simulink model "GRM_Airframe"  (R2018b)
settings: Solver=FixedStepAuto  StartTime=0.0  StopTime=T_sim  FixedStep=0.001  RelTol=1e-3
PreLoadFcn:
  | addpath('init_functions');
  | init_grm;
  | addpath('parameters');
  | para_def_grm;
values from neighbouring files (symbols this model uses):
  act_dmp = 0.6322    [para_def_grm.m]
  act_omega = 59.9250    (= 59.925)    [para_def_grm.m]
  aero = load('aero.mat')    [para_def_grm.m]
  c_be = -6.5e-3    (= -0.0065)    [init_grm.m]
  c_h_geop0 = 0    [init_grm.m]
  c_h_geope = 11e3    (= 11000)    [init_grm.m]
  c_pa0 = 101325    [init_grm.m]
  c_pe = -c_g0/c_be/sgc    (= 5.25587981272)    [init_grm.m]
  c_r0 = 6371000.79    [init_grm.m]
  c_rot = 7.292115e-5    (= 7.292115e-05)    [init_grm.m]
  c_Tmp0 = 288.15    [init_grm.m]
  d_siB_0 = 0    [para_def_grm.m]
  d_siB_max = deg2rad(1200)    [para_def_grm.m]
  d_siB_min = deg2rad(-1200)    [para_def_grm.m]
  dd_siB_max = deg2rad(50000)    [para_def_grm.m]
  dd_siB_min = deg2rad(-50000)    [para_def_grm.m]
  de_JBBB_xx = JBBB_xx_0 - JBBB_xx_e    (= 0)    [para_def_grm.m]
  de_JBBB_yy = JBBB_yy_0 - JBBB_yy_e    (= 0)    [para_def_grm.m]
  de_JBBB_zz = JBBB_zz_0 - JBBB_zz_e    (= 0)    [para_def_grm.m]
  de_mM = m_fuel_lookup(end)    [para_def_grm.m]
  F_prp = [450.52;428.7;423.25;391.61;352.34;304.35;266.17;243.26;216.92 ... (first row only)    [para_def_grm.m]
  flag_I_aero_switch = 1    [init_grm.m]
  flag_I_flat = 1    [init_grm.m]
  flag_I_gravity_switch = 1    [init_grm.m]
  flag_I_rot = 0    [init_grm.m]
  hcr = 1.4    [init_grm.m]
  J0PB_e = TBP*J0PP_e*TBP'    [para_def_grm.m]
  JMMM_0 = TBP*J0PP_0*TBP'    [para_def_grm.m]
  JMMM_e = TBP*J0PP_e*TBP'    [para_def_grm.m]
  lat_0 = 0    [init_grm.m]
  lon_0 = 0    [init_grm.m]
  m0 = mB_0    (= 3.30977)    [para_def_grm.m]
  m_fuel_lookup = [0;0.0573;0.1127;0.1667;0.2186;0.2681;0.3149;0.3588 ... (first row only)    [para_def_grm.m]
  mB_0 = 3.30977    [para_def_grm.m]
  mM_0 = 1.119    [para_def_grm.m]
  mM_e = de_mM    [para_def_grm.m]
  p0PB = [x0PB;y0PB;z0PB]    [para_def_grm.m]
  pBII_0 = TIE_0*pBEE_0    [init_grm.m]
  pMPB = [xMPB;yMPB;zMPB]    [para_def_grm.m]
  pNPB = [0;0;0]    [para_def_grm.m]
  qEG_0 = q12_from_T12(TEG)    [init_grm.m]
  qIB_0 = qumul(qIG_0,qGB_0)    [init_grm.m]
  qIE_0 = q12_from_T12(TIE_0)    [init_grm.m]
  sgc = 287.05287    [init_grm.m]
  siB_0 = 0    [para_def_grm.m]
  siB_max = deg2rad(30)    [para_def_grm.m]
  siB_min = deg2rad(-30)    [para_def_grm.m]
  t_prp1 = [0.04;0.28;0.54;1;1.48;1.99;2.51;3;3.5;3.67;3.82;4]    [para_def_grm.m]
  t_prp2 = t_prp2'    [para_def_grm.m]
  Tr3r4 = [1,1,1,1;1,1,-1,-1;-1,1,1,-1]*0.25    [para_def_grm.m]
  tRRR = 0    [para_def_grm.m]
  unc_act_bl = 0    [para_def_grm.m]
  unc_act_off = 0    [para_def_grm.m]
  unc_act_scale = 1    [para_def_grm.m]
  unc_aero_Cl_scale = 1    [para_def_grm.m]
  unc_aero_Cm_scale = 1    [para_def_grm.m]
  unc_aero_Cn_scale = 1    [para_def_grm.m]
  unc_aero_Cx_scale = 1    [para_def_grm.m]
  unc_aero_Cy_scale = 1    [para_def_grm.m]
  unc_aero_Cz_scale = 1    [para_def_grm.m]
  unc_cg_x = 0    [para_def_grm.m]
  unc_cg_y = 0    [para_def_grm.m]
  unc_cg_z = 0    [para_def_grm.m]
  unc_mB_bl = 0    [para_def_grm.m]
  unc_mB_scale = 1    [para_def_grm.m]
  unc_moi_Jxx = 0    [para_def_grm.m]
  unc_moi_Jyy = 0    [para_def_grm.m]
  unc_moi_Jzz = 0    [para_def_grm.m]
  unc_prp_scale = 1    [para_def_grm.m]
  unc_prp_x = 0    [para_def_grm.m]
  unc_prp_y = 0    [para_def_grm.m]
  unc_prp_z = 0    [para_def_grm.m]
  vBII_0 = vBEE_0 + cross(wIEI_0,pBII_0)    [init_grm.m]
  wBIB_0 = r2_from_r1_trans_q21(wBII_0,qBI_0)    [init_grm.m]
  x0PB = -0.5    [para_def_grm.m]
  xMPB = -0.9    [para_def_grm.m]
  y0PB = 0    [para_def_grm.m]
  yMPB = 0    [para_def_grm.m]
  z0PB = 0    [para_def_grm.m]
  zMPB = 0    [para_def_grm.m]
undefined symbols (not defined in the file or in its folder): c_b_WGS, c_flat, c_grav, c_rsma, d_mB_lookup, t_dmB
libraries: simulink_extras x11, simulink x3
(part 1 of 6)
settings Model: Creator=ga97lot  LastModifiedBy=ga97lot

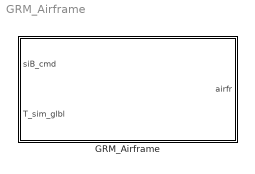
== system GRM_Airframe ==
  GRM_Airframe : Subsystem
      mask Display: image('H:\Sicherung Semesterarbeit\CAD\grm_2.png');

== system GRM_Airframe/GRM_Airframe ==
  siB_cmd : Inport
  T_sim_glbl : Inport  Port=2
  Bus Creator : BusCreator  Inputs=8
  aerodynamics : Subsystem
  environment : Subsystem
  fin_actuators : Subsystem
  forces_moments : Subsystem
  gravity : Subsystem
  input : Subsystem
  motion_kinematics : Subsystem
  propulsion : Subsystem
  rb_eom : Subsystem
  stream_flow : Subsystem
  weight_and_balance : Subsystem
  airfr : Outport
  wires:
  [fin] -> Bus Creator/7
  [motion_kin] -> Bus Creator/6
  [str_flow] -> Bus Creator/5
  [aero] -> Bus Creator/4
  [grav] -> Bus Creator/3
  [prp] -> Bus Creator/8
  [motion_kin] -> rb_eom/1(mot_kin)
  [prp] -> forces_moments/4(prp)
  [motion_kin] -> forces_moments/2(motion_kin)
  Bus Creator/1 -> airfr/1  "airfr_bus"
  [wab] -> Bus Creator/2
  input/1(cmd_bus) -> fin_actuators/1(cmd)
  siB_cmd/1 -> input/1(siB_cmd)
  aerodynamics/1(aero) -> [aero], forces_moments/1(aero)
  forces_moments/1(for_mom_bus) -> rb_eom/2(for_mom)
  stream_flow/1(str_flow) -> [str_flow], aerodynamics/1(str_flow)
  [wab] -> propulsion/2(wab)
  weight_and_balance/1(wab) -> gravity/2(wab), rb_eom/3(wab), [wab]
  T_sim_glbl/1 -> propulsion/1(env_glbl), environment/2(env_glbl), [env_glbl]
  gravity/1(grav) -> forces_moments/3(grav), [grav]
  [env_glbl] -> aerodynamics/4(env_glbl)
  fin_actuators/1(fin) -> aerodynamics/2(fin), [fin]
  [env_glbl] -> weight_and_balance/2(env_glb)
  [wab] -> aerodynamics/3(wab)
  motion_kinematics/1(motion_kin) -> [motion_kin], stream_flow/2(motion_kin)
  propulsion/1(prp) -> [prp], weight_and_balance/1(prp)
  environment/1(env) -> stream_flow/3(env), gravity/1(env)
  rb_eom/1(flight_dyn) -> Bus Creator/1, motion_kinematics/1(flight_dyn), environment/1(flight_dyn), stream_flow/1(flight_dyn)

== system GRM_Airframe/GRM_Airframe/aerodynamics ==
  str_flow : Inport
  fin : Inport  Port=2
  wab : Inport  Port=3
  env_glbl : Inport  Port=4
  Bus Selector : BusSelector  OutputSignals=qdynB,MaB,alB,beB,hBE,wBIB_star
  Bus Selector1 : BusSelector  OutputSignals=afinB
  Bus Selector2 : BusSelector  OutputSignals=pBSB
  aerodynamic_via_lookup : Subsystem
  logic_base_drag : Subsystem
  aero : Outport
  wires:
  logic_base_drag/1(flag_base_drag) -> aerodynamic_via_lookup/9(flag_I_prp)
  env_glbl/1 -> logic_base_drag/1(env_glbl)
  aerodynamic_via_lookup/1(aero_bus) -> aero/1
  Bus Selector/6 -> aerodynamic_via_lookup/7(wBIB_star)  "<wBIB_star>"
  Bus Selector1/1 -> aerodynamic_via_lookup/8(afinB)  "<afinB>"
  Bus Selector/5 -> aerodynamic_via_lookup/6(hBE)  "<hBE>"
  Bus Selector/4 -> aerodynamic_via_lookup/5(beB)  "<beB>"
  Bus Selector/3 -> aerodynamic_via_lookup/4(alB)  "<alB>"
  Bus Selector/2 -> aerodynamic_via_lookup/3(MaB)  "<MaB>"
  Bus Selector/1 -> aerodynamic_via_lookup/2(qdynB)  "<qdynB>"
  Bus Selector2/1 -> aerodynamic_via_lookup/1(pBSB)  "<pBSB>"
  fin/1 -> Bus Selector1/1
  wab/1 -> Bus Selector2/1
  str_flow/1 -> Bus Selector/1

== system GRM_Airframe/GRM_Airframe/environment ==
  flight_dyn : Inport
  env_glbl : Inport  Port=2
  Bus Creator1 : BusCreator  Inputs=2
  Bus Creator2 : BusCreator  Inputs=2
  Bus Selector : BusSelector  OutputSignals=lon,lat,hBE
  Bus Selector1 : BusSelector  OutputSignals=atm_dyn_bus
  Saturation : Saturate  UpperLimit=inf  LowerLimit=eps
      settings: AttributesFormatString=|
      | %<UpperLimit>
      | %<LowerLimit>
  WGS84_Gravitation : Subsystem  mask{flg_omega_enabled=on}
      mask prompts: flg_omega_enabled "Zentripetalbeschleunigung mitberechnen"
      mask help:
      | Dieser Block berechnet die Gravitation für das idealisierte WGS84
      | Ellipsoid. Die Berechnung ist hierbei nach dem Technical Report
      | "Department of Defense World Geodetic System 1984", NIMA TR8350.2,
      | Third Edition, Amendment 1 vom 3 Januar 2000 implementiert.
      | Das Modell ist gültig für alle Höhen über dem WGS84 Referenzellipsoid, und
      | ist somit der reinen Taylorexpansion des Somigliana Modells überlegen
      | (siehe Kapitel 4.3 des WGS84 reports).
      |
      | ---------------------------------------------------------------------------
      | Longitude [rad]: Nach WGS84 definierte Geodätische Länge.  (lambda)
      | Lattitude [rad]: Nach WGS84 definierte Geodätische Breite. (phi)
      | Height [m]: Höhe über dem WGS84 Referenzellipsoid.
      mask init:
      | [ c_rsma, c_b_WGS, c_grav, c_rot] = init_WGS84_Gravitationsmodell();
  atmosphere_static_ISO_2533 : Subsystem
  convert_to_local_frame : Subsystem
  env : Outport
  wires:
  Bus Selector1/1 -> Bus Creator1/2  "<atm_dyn_bus>"
  env_glbl/1 -> atmosphere_static_ISO_2533/2(env_glbl), Bus Selector1/1
  atmosphere_static_ISO_2533/1(atm_stat) -> Bus Creator1/1  "atm_stat_bus"
  Saturation/1 -> WGS84_Gravitation/3(h)
  Bus Creator1/1 -> Bus Creator2/2  "atm_bus"
  Bus Selector/2 -> WGS84_Gravitation/2(lat)  "<lat>"
  Bus Creator2/1 -> env/1  "env_bus"
  Bus Selector/3 -> Saturation/1, atmosphere_static_ISO_2533/1(hBE)  "<hBE>"
  Bus Selector/1 -> WGS84_Gravitation/1(lon)  "<lon>"
  WGS84_Gravitation/1(gE) -> convert_to_local_frame/1(gE)
  flight_dyn/1 -> Bus Selector/1
  convert_to_local_frame/1(gBG) -> Bus Creator2/1

== system GRM_Airframe/GRM_Airframe/fin_actuators ==
  cmd : Inport
  Bus Creator3 : BusCreator  Inputs=7
  Bus Selector : BusSelector  OutputSignals=siB_cmd
  Constant7 : Constant  Value=tRRR
  Demux : Demux
  Rudder : Subsystem  mask{siB_max=siB_max, siB_min=siB_min, d_siB_max=d_siB_max, d_siB_min=d_siB_min, dd_siB_max=dd_siB_max, dd_siB_min=dd_siB_min, omega=act_omega, dmp=act_dmp, unc_bl=unc_act_bl, unc_scale=unc_act_scale, unc_off=unc_act_off, siB_0=siB_0, d_siB_0=d_siB_0}
      mask prompts: siB_max "Obere Limitierung des Ruderstellwinkels in [rad]"; siB_min "Untere Limitierung des Ruderstellwinkels in [rad]"; d_siB_max "Obere Limitierung der Ruderstellwinkelgeschwindigkeit in [rad/s]"; d_siB_min "Untere Limitierung der Ruderstellwinkelgeschwindigkeit in [rad/s]"; dd_siB_max "Obere Limitierung der Ruderstellwinkelbeschleunigung in [rad/s^2]"; dd_siB_min "Untere Limitierung der Ruderstellwinkelbeschleunigung in [rad/s^2]"; omega "Eckfrequenz in [Hz]"; dmp "Dämpfung in [kg/s]"; unc_bl "Rückschlag des Aktuators (Backlash) in [rad]"; unc_scale "Skalenfehler in [-]"; unc_off "Versatz (Offset) in [rad]"; siB_0 "Startwert Ruderwinkel in [rad]"; d_siB_0 "Startwert Ruderwinkelgeschwindigkeiten in [rad/s]"
      mask DialogControl ParameterGroupVar Prompt: Limitierungen
      mask DialogControl Container3 Prompt: Dynamik
      mask DialogControl Container4 Prompt: Aktuatorfehler
      mask DialogControl Container5 Prompt: Startwerte
  Rudder1 : Subsystem  mask{siB_max=siB_max, siB_min=siB_min, d_siB_max=d_siB_max, d_siB_min=d_siB_min, dd_siB_max=dd_siB_max, dd_siB_min=dd_siB_min, omega=act_omega, dmp=act_dmp, unc_bl=unc_act_bl, unc_scale=unc_act_scale, unc_off=unc_act_off, siB_0=siB_0, d_siB_0=d_siB_0}
      mask prompts: siB_max "Obere Limitierung des Ruderstellwinkels in [rad]"; siB_min "Untere Limitierung des Ruderstellwinkels in [rad]"; d_siB_max "Obere Limitierung der Ruderstellwinkelgeschwindigkeit in [rad/s]"; d_siB_min "Untere Limitierung der Ruderstellwinkelgeschwindigkeit in [rad/s]"; dd_siB_max "Obere Limitierung der Ruderstellwinkelbeschleunigung in [rad/s^2]"; dd_siB_min "Untere Limitierung der Ruderstellwinkelbeschleunigung in [rad/s^2]"; omega "Eckfrequenz in [Hz]"; dmp "Dämpfung in [kg/s]"; unc_bl "Rückschlag des Aktuators (Backlash) in [rad]"; unc_scale "Skalenfehler in [-]"; unc_off "Versatz (Offset) in [rad]"; siB_0 "Startwert Ruderwinkel in [rad]"; d_siB_0 "Startwert Ruderwinkelgeschwindigkeiten in [rad/s]"
      mask DialogControl ParameterGroupVar Prompt: Limitierungen
      mask DialogControl Container3 Prompt: Dynamik
      mask DialogControl Container4 Prompt: Aktuatorfehler
      mask DialogControl Container5 Prompt: Startwerte
  Rudder2 : Subsystem  mask{siB_max=siB_max, siB_min=siB_min, d_siB_max=d_siB_max, d_siB_min=d_siB_min, dd_siB_max=dd_siB_max, dd_siB_min=dd_siB_min, omega=act_omega, dmp=act_dmp, unc_bl=unc_act_bl, unc_scale=unc_act_scale, unc_off=unc_act_off, siB_0=siB_0, d_siB_0=d_siB_0}
      mask prompts: siB_max "Obere Limitierung des Ruderstellwinkels in [rad]"; siB_min "Untere Limitierung des Ruderstellwinkels in [rad]"; d_siB_max "Obere Limitierung der Ruderstellwinkelgeschwindigkeit in [rad/s]"; d_siB_min "Untere Limitierung der Ruderstellwinkelgeschwindigkeit in [rad/s]"; dd_siB_max "Obere Limitierung der Ruderstellwinkelbeschleunigung in [rad/s^2]"; dd_siB_min "Untere Limitierung der Ruderstellwinkelbeschleunigung in [rad/s^2]"; omega "Eckfrequenz in [Hz]"; dmp "Dämpfung in [kg/s]"; unc_bl "Rückschlag des Aktuators (Backlash) in [rad]"; unc_scale "Skalenfehler in [-]"; unc_off "Versatz (Offset) in [rad]"; siB_0 "Startwert Ruderwinkel in [rad]"; d_siB_0 "Startwert Ruderwinkelgeschwindigkeiten in [rad/s]"
      mask DialogControl ParameterGroupVar Prompt: Limitierungen
      mask DialogControl Container3 Prompt: Dynamik
      mask DialogControl Container4 Prompt: Aktuatorfehler
      mask DialogControl Container5 Prompt: Startwerte
  Rudder3 : Subsystem  mask{siB_max=siB_max, siB_min=siB_min, d_siB_max=d_siB_max, d_siB_min=d_siB_min, dd_siB_max=dd_siB_max, dd_siB_min=dd_siB_min, omega=act_omega, dmp=act_dmp, unc_bl=unc_act_bl, unc_scale=unc_act_scale, unc_off=unc_act_off, siB_0=siB_0, d_siB_0=d_siB_0}
      mask prompts: siB_max "Obere Limitierung des Ruderstellwinkels in [rad]"; siB_min "Untere Limitierung des Ruderstellwinkels in [rad]"; d_siB_max "Obere Limitierung der Ruderstellwinkelgeschwindigkeit in [rad/s]"; d_siB_min "Untere Limitierung der Ruderstellwinkelgeschwindigkeit in [rad/s]"; dd_siB_max "Obere Limitierung der Ruderstellwinkelbeschleunigung in [rad/s^2]"; dd_siB_min "Untere Limitierung der Ruderstellwinkelbeschleunigung in [rad/s^2]"; omega "Eckfrequenz in [Hz]"; dmp "Dämpfung in [kg/s]"; unc_bl "Rückschlag des Aktuators (Backlash) in [rad]"; unc_scale "Skalenfehler in [-]"; unc_off "Versatz (Offset) in [rad]"; siB_0 "Startwert Ruderwinkel in [rad]"; d_siB_0 "Startwert Ruderwinkelgeschwindigkeiten in [rad/s]"
      mask DialogControl ParameterGroupVar Prompt: Limitierungen
      mask DialogControl Container3 Prompt: Dynamik
      mask DialogControl Container4 Prompt: Aktuatorfehler
      mask DialogControl Container5 Prompt: Startwerte
  Vector Concatenate1 : Concatenate  NumInputs=4
  Vector Concatenate2 : Concatenate  NumInputs=4
  Vector Concatenate3 : Concatenate  NumInputs=4
  control_allocation : Subsystem
  fin : Outport
  wires:
  control_allocation/4(dd_finB) -> Bus Creator3/5
  control_allocation/3(d_finB) -> Bus Creator3/4
  control_allocation/2(finB) -> Bus Creator3/3
  control_allocation/1(Tr3r4) -> Bus Creator3/2
  Vector Concatenate3/1 -> control_allocation/3(dd_siB), Bus Creator3/6  "dd_siB"
  Vector Concatenate2/1 -> control_allocation/2(d_siB), Bus Creator3/7  "d_siB"
  Vector Concatenate1/1 -> control_allocation/1(siB), Bus Creator3/1  "siB"
  Bus Creator3/1 -> fin/1  "fin_bus"
  Rudder/1(siB) -> Vector Concatenate1/1
  Rudder/3(dd_siB) -> [dd_siB1]
  Demux/2 -> Rudder1/1(siB_c)
  Rudder2/3(dd_siB) -> [dd_siB3]
  Rudder/2(d_siB) -> [d_siB1]
  Rudder3/3(dd_siB) -> [dd_siB4]
  Rudder1/3(dd_siB) -> [dd_siB2]
  Rudder1/1(siB) -> Vector Concatenate1/2
  [dd_siB1] -> Vector Concatenate3/1
  cmd/1 -> Bus Selector/1
  [dd_siB3] -> Vector Concatenate3/3
  [dd_siB4] -> Vector Concatenate3/4
  Demux/1 -> Rudder/1(siB_c)
  Rudder3/2(d_siB) -> [d_siB4]
  Demux/3 -> Rudder2/1(siB_c)
  [dd_siB2] -> Vector Concatenate3/2
  Constant7/1 -> Rudder/2(tRRR), Rudder2/2(tRRR), Rudder3/2(tRRR), Rudder1/2(tRRR)
  [d_siB2] -> Vector Concatenate2/2
  Bus Selector/1 -> Demux/1  "<siB_cmd>"
  [d_siB1] -> Vector Concatenate2/1
  [d_siB4] -> Vector Concatenate2/4
  Rudder2/1(siB) -> Vector Concatenate1/3
  Rudder1/2(d_siB) -> [d_siB2]
  Rudder3/1(siB) -> Vector Concatenate1/4
  Rudder2/2(d_siB) -> [d_siB3]
  Demux/4 -> Rudder3/1(siB_c)
  [d_siB3] -> Vector Concatenate2/3

== system GRM_Airframe/GRM_Airframe/forces_moments ==
  aero : Inport
  motion_kin : Inport  Port=2
  grav : Inport  Port=3
  prp : Inport  Port=4
  Add : Sum  Inputs=+++
  Add1 : Sum
  Bus Creator : BusCreator  Inputs=2
  Bus Selector : BusSelector  OutputSignals=FBAB,MBAB
  Bus Selector1 : BusSelector  OutputSignals=TGB
  Bus Selector2 : BusSelector  OutputSignals=FBGG
  Bus Selector3 : BusSelector  OutputSignals=FBPB,MBPB
  Math Function : Math  Operator=transpose  SaturateOnIntegerOverflow=on
  Product : Product  Multiplication=Matrix(*)
  for_mom_bus : Outport
  wires:
  Bus Selector3/2 -> Add1/2  "<MBPB>"
  Bus Creator/1 -> for_mom_bus/1  "for_mom_bus"
  Bus Selector3/1 -> Add/3  "<FBPB>"
  Bus Selector/2 -> Add1/1  "<MBAB>"
  Add1/1 -> Bus Creator/2  "MBTB"
  grav/1 -> Bus Selector2/1
  Add/1 -> Bus Creator/1  "FBTB"
  motion_kin/1 -> Bus Selector1/1
  prp/1 -> Bus Selector3/1
  Product/1 -> Add/2  "FBGB"
  aero/1 -> Bus Selector/1
  Math Function/1 -> Product/1  "TBG"
  Bus Selector1/1 -> Math Function/1  "<TGB>"
  Bus Selector2/1 -> Product/2  "<FBGG>"
  Bus Selector/1 -> Add/1  "<FBAB>"

== system GRM_Airframe/GRM_Airframe/gravity ==
  env : Inport
  wab : Inport  Port=2
  Bus Creator3 : BusCreator  Inputs=1
  Bus Selector : BusSelector  OutputSignals=gBG,atm_bus.atm_stat_bus.hBE
  Bus Selector1 : BusSelector  OutputSignals=mB
  Product : Product
  launch_rail : Subsystem
  grav : Outport
  wires:
  env/1 -> Bus Selector/1
  Bus Selector1/1 -> Product/2  "<mB>"
  wab/1 -> Bus Selector1/1
  Bus Creator3/1 -> grav/1  "grav_bus"
  Product/1 -> Bus Creator3/1  "FBGG"
  Bus Selector/1 -> launch_rail/1(gBG_c)  "<gBG>"
  Bus Selector/2 -> launch_rail/2(hBE)  "<hBE>"
  launch_rail/1(gBG) -> Product/1

== system GRM_Airframe/GRM_Airframe/input ==
  siB_cmd : Inport
  Bus Creator2 : BusCreator  Inputs=1
  cmd_bus : Outport
  wires:
  Bus Creator2/1 -> cmd_bus/1  "cmd_bus"
  siB_cmd/1 -> Bus Creator2/1

== system GRM_Airframe/GRM_Airframe/motion_kinematics ==
  flight_dyn : Inport
  Bus Creator : BusCreator  Inputs=7
  Bus Selector : BusSelector  OutputSignals=lat,lon,qIB
  calc_motion_kinematics : Subsystem
  motion_kin : Outport
  wires:
  calc_motion_kinematics/7(TIB) -> Bus Creator/7
  calc_motion_kinematics/6(wEGG) -> Bus Creator/6
  calc_motion_kinematics/5(TEG) -> Bus Creator/5
  calc_motion_kinematics/4(TGB) -> Bus Creator/4
  calc_motion_kinematics/3(TEB) -> Bus Creator/3
  calc_motion_kinematics/2(TIE) -> Bus Creator/2
  calc_motion_kinematics/1(wIEE) -> Bus Creator/1
  Bus Selector/3 -> calc_motion_kinematics/3(qIB)  "<qIB>"
  Bus Selector/2 -> calc_motion_kinematics/2(lon)  "<lon>"
  Bus Selector/1 -> calc_motion_kinematics/1(lat)  "<lat>"
  Bus Creator/1 -> motion_kin/1  "motion_kin_bus"
  flight_dyn/1 -> Bus Selector/1

== system GRM_Airframe/GRM_Airframe/propulsion ==
  env_glbl : Inport
  wab : Inport  Port=2
  Bus Creator1 : BusCreator  Inputs=3
  prp_look_up : Subsystem
  prp_uncertainty : Subsystem
  prp : Outport
  wires:
  prp_look_up/1(dmB) -> Bus Creator1/1
  wab/1 -> prp_uncertainty/2(wab)
  prp_uncertainty/1(FBPB) -> Bus Creator1/2
  prp_uncertainty/2(MBPB) -> Bus Creator1/3
  env_glbl/1 -> prp_look_up/1(env_glbl_bus)
  prp_look_up/2(FBPM) -> prp_uncertainty/1(FBPM)
  Bus Creator1/1 -> prp/1  "prp_bus"

== system GRM_Airframe/GRM_Airframe/rb_eom ==
  mot_kin : Inport
  for_mom : Inport  Port=2
  wab : Inport  Port=3
  Bus Creator : BusCreator  Inputs=12
  calc_bus_flight_dyn_bus_entries : Subsystem
  eom_6dof : Subsystem
  flight_dyn : Outport
  wires:
  calc_bus_flight_dyn_bus_entries/12(vBIB) -> Bus Creator/12
  calc_bus_flight_dyn_bus_entries/11(euIB) -> Bus Creator/11
  calc_bus_flight_dyn_bus_entries/10(pBII) -> Bus Creator/10
  eom_6dof/1(eom) -> calc_bus_flight_dyn_bus_entries/2(eom)
  wab/1 -> eom_6dof/2(wab)
  for_mom/1 -> eom_6dof/1(for_mom)
  Bus Creator/1 -> flight_dyn/1  "flight_dyn_bus"
  calc_bus_flight_dyn_bus_entries/9(d_vBII) -> Bus Creator/9
  calc_bus_flight_dyn_bus_entries/8(d_wBIB) -> Bus Creator/8
  calc_bus_flight_dyn_bus_entries/7(wBIB) -> Bus Creator/7
  calc_bus_flight_dyn_bus_entries/6(qIB) -> Bus Creator/6
  calc_bus_flight_dyn_bus_entries/5(vBII) -> Bus Creator/5
  calc_bus_flight_dyn_bus_entries/4(hBE) -> Bus Creator/4
  calc_bus_flight_dyn_bus_entries/3(lat) -> Bus Creator/3
  calc_bus_flight_dyn_bus_entries/2(lon) -> Bus Creator/2
  calc_bus_flight_dyn_bus_entries/1(aBIB) -> Bus Creator/1
  mot_kin/1 -> calc_bus_flight_dyn_bus_entries/1(mot_kin)

== system GRM_Airframe/GRM_Airframe/stream_flow ==
  flight_dyn : Inport
  motion_kin : Inport  Port=2
  env : Inport  Port=3
  Bus Selector1 : BusSelector  OutputSignals=atm_bus.atm_stat_bus.rho,atm_bus.atm_stat_bus.sos,atm_bus.atm_stat_bus.hBE,atm_bus.atm_dyn_bus.vWEG
  Bus Selector2 : BusSelector  OutputSignals=vBII,pBII,wBIB
  Bus Selector3 : BusSelector  OutputSignals=TIB,wIEE,TIE,TGB
  calc_stream_flow : Subsystem
  str_flow : Outport
  wires:
  Bus Selector3/4 -> calc_stream_flow/4(TGB)  "<TGB>"
  Bus Selector1/4 -> calc_stream_flow/11(vWEG)  "<vWEG>"
  Bus Selector2/2 -> calc_stream_flow/6(pBII)  "<pBII>"
  calc_stream_flow/1(str_flow) -> str_flow/1
  Bus Selector1/3 -> calc_stream_flow/10(hBE)  "<hBE>"
  Bus Selector1/2 -> calc_stream_flow/9(sos)  "<sos>"
  Bus Selector1/1 -> calc_stream_flow/8(rho)  "<rho>"
  Bus Selector2/3 -> calc_stream_flow/7(wBIB)  "<wBIB>"
  Bus Selector2/1 -> calc_stream_flow/5(vBII)  "<vBII>"
  Bus Selector3/3 -> calc_stream_flow/3(TIE)  "<TIE>"
  Bus Selector3/2 -> calc_stream_flow/2(wIEE)  "<wIEE>"
  Bus Selector3/1 -> calc_stream_flow/1(TIB)  "<TIB>"
  env/1 -> Bus Selector1/1
  flight_dyn/1 -> Bus Selector2/1
  motion_kin/1 -> Bus Selector3/1

== system GRM_Airframe/GRM_Airframe/weight_and_balance ==
  prp : Inport
  env_glb : Inport  Port=2
  Bus Creator1 : BusCreator  Inputs=4
  Bus Selector2 : BusSelector  OutputSignals=T_sim_glbl,T_sim_lnch
  Subtract : Sum  Inputs=+-
  center_of_gravity : Subsystem
  d_moi : Subsystem
  mass : Subsystem
  mass_uncertainty : Subsystem
  moi : Subsystem
  wab : Outport
  wires:
  d_moi/1(d_JBBB) -> Bus Creator1/4
  prp/1 -> d_moi/1(prp)
  Subtract/1 -> mass/1(sim_time_launch)
  mass/1(mB_c) -> mass_uncertainty/1(mB_c)
  mass_uncertainty/1(mB) -> Bus Creator1/1, center_of_gravity/1(mB)
  mass/2(mM) -> center_of_gravity/2(mM), moi/2(mM)
  moi/1(JBBB) -> Bus Creator1/3
  center_of_gravity/1(pBSB) -> Bus Creator1/2, moi/1(pBPB)
  Bus Creator1/1 -> wab/1  "wab_bus"
  env_glb/1 -> Bus Selector2/1
  Bus Selector2/1 -> Subtract/1  "<T_sim_glbl>"
  Bus Selector2/2 -> Subtract/2  "<T_sim_lnch>"

== system GRM_Airframe/GRM_Airframe/aerodynamics/aerodynamic_via_lookup ==
  pBSB : Inport
  qdynB : Inport  Port=2
  MaB : Inport  Port=3
  alB : Inport  Port=4
  beB : Inport  Port=5
  hBE : Inport  Port=6
  wBIB_star : Inport  Port=7
  afinB : Inport  Port=8
  flag_I_prp : Inport  Port=9
  Bus Creator : BusCreator  Inputs=2
  calc_aero_coefficients : Subsystem
  calc_aero_for_mom : Subsystem
  calc_derivatives : Subsystem
  transform_rad2deg_al_be : Subsystem
  transform_rad2deg_fin : Subsystem
  transform_rad2deg_rates : Subsystem
  aero_bus : Outport
  wires:
  transform_rad2deg_al_be/2(beB_deg) -> calc_derivatives/4(beB)
  transform_rad2deg_al_be/1(alB_deg) -> calc_derivatives/3(alB)
  beB/1 -> transform_rad2deg_al_be/2(beB)
  afinB/1 -> transform_rad2deg_fin/1(afinB)
  qdynB/1 -> calc_aero_for_mom/3(qdynB)
  calc_aero_for_mom/2(MBAB) -> Bus Creator/2
  calc_aero_coefficients/6(Cn) -> calc_aero_for_mom/9(Cn)
  calc_aero_coefficients/1(Cx) -> calc_aero_for_mom/4(Cx)
  calc_aero_coefficients/5(Cm) -> calc_aero_for_mom/8(Cm)
  calc_derivatives/4(Cl_deriv) -> calc_aero_coefficients/4(Cl_deriv)
  calc_aero_coefficients/3(Cz) -> calc_aero_for_mom/6(Cz)
  hBE/1 -> calc_aero_for_mom/1(hBE), calc_derivatives/1(hBE)
  flag_I_prp/1 -> calc_aero_coefficients/13(flag_base_drag)
  calc_derivatives/6(Cn_deriv) -> calc_aero_coefficients/6(Cn_deriv)
  wBIB_star/1 -> transform_rad2deg_rates/1(wBIB_star)
  calc_derivatives/3(Cz_deriv) -> calc_aero_coefficients/3(Cz_deriv)
  pBSB/1 -> calc_aero_for_mom/2(pBSB)
  transform_rad2deg_rates/2(qBIB_star_deg) -> calc_aero_coefficients/11(qBIB_star)
  transform_rad2deg_rates/3(rBIB_star_deg) -> calc_aero_coefficients/12(rBIB_star)
  Bus Creator/1 -> aero_bus/1  "aero_bus"
  calc_aero_coefficients/2(Cy) -> calc_aero_for_mom/5(Cy)
  calc_derivatives/5(Cm_deriv) -> calc_aero_coefficients/5(Cm_deriv)
  calc_derivatives/2(Cy_deriv) -> calc_aero_coefficients/2(Cy_deriv)
  transform_rad2deg_rates/1(pBIB_star_deg) -> calc_aero_coefficients/10(pBIB_star)
  transform_rad2deg_fin/3(xiB_deg) -> calc_aero_coefficients/9(xiB_deg)
  transform_rad2deg_fin/2(zeB_deg) -> calc_aero_coefficients/8(zeB_deg), calc_derivatives/6(zeB_deg)
  alB/1 -> transform_rad2deg_al_be/1(alB)
  transform_rad2deg_fin/1(etB_deg) -> calc_derivatives/5(etB_deg), calc_aero_coefficients/7(etB_deg)
  calc_derivatives/1(Cx_deriv) -> calc_aero_coefficients/1(Cx_deriv)
  calc_aero_for_mom/1(FBAB) -> Bus Creator/1
  MaB/1 -> calc_derivatives/2(MaB)
  calc_aero_coefficients/4(Cl) -> calc_aero_for_mom/7(Cl)

== system GRM_Airframe/GRM_Airframe/aerodynamics/logic_base_drag ==
  env_glbl : Inport
  Bus Selector1 : BusSelector  OutputSignals=T_sim_glbl,T_sim_lnch
  Constant : Constant  Value=t_prp2(end)
  MATLAB Function : MATLAB Function  TreatAsAtomicUnit=on
  Subtract : Sum  Inputs=+-
  flag_base_drag : Outport
  wires:
  env_glbl/1 -> Bus Selector1/1
  Bus Selector1/2 -> Subtract/2  "<T_sim_lnch>"
  Bus Selector1/1 -> Subtract/1  "<T_sim_glbl>"
  MATLAB Function/1(flag_base_drag) -> flag_base_drag/1  "flag_base_drag"
  Constant/1 -> MATLAB Function/2(t_prp2)
  Subtract/1 -> MATLAB Function/1(u)

== system GRM_Airframe/GRM_Airframe/environment/WGS84_Gravitation ==
  lon : Inport  PortDimensions=1
  lat : Inport  Port=2  PortDimensions=1
  h : Inport  Port=3  PortDimensions=1
  Assertion : Assertion  AssertionFailFcn="error('WGS84 Gravitationsmodell: Die Werte des Eingangs \"h\" muessen groesser als 0 sein')"
  Assertion1 : Assertion  AssertionFailFcn="error('WGS84 Gravitationsmodell: Die Werte des Eingangs \"Long\" muessen zwischen -180 und +180 liegen')"
  Assertion2 : Assertion  AssertionFailFcn="error('WGS84 Gravitationsmodell: Die Werte des Eingangs \"Lat\" muessen zwischen -90 und +90 liegen')"
  Compare To Constant : simulink/Logic and Bit Operations/Compare To Constant  relop=>=  const=0  OutDataTypeStr=boolean
      settings: SourceProductName=ISim Simulink Block Set
  Interval Test : simulink/Logic and Bit Operations/Interval Test  IntervalClosedRight=on  uplimit=pi  IntervalClosedLeft=on  lowlimit=-pi  OutDataTypeStr=boolean
      settings: SourceProductName=ISim Simulink Block Set
  Interval Test1 : simulink/Logic and Bit Operations/Interval Test  IntervalClosedRight=on  uplimit=pi/2  IntervalClosedLeft=on  lowlimit=-pi/2  OutDataTypeStr=boolean
      settings: SourceProductName=ISim Simulink Block Set
  WGS84_2_ECEF : Subsystem
  WGS84_Gravity_Implementation : MATLAB Function  TreatAsAtomicUnit=on
  gE : Outport  PortDimensions=3
  wires:
  WGS84_Gravity_Implementation/1(gamma_R) -> gE/1  "gE"
  h/1 -> Compare To Constant/1, WGS84_2_ECEF/1(h)  "h"
  lon/1 -> WGS84_2_ECEF/2(lon), Interval Test/1, WGS84_Gravity_Implementation/3(long_rad)  "lon"
  lat/1 -> WGS84_2_ECEF/3(lat), Interval Test1/1, WGS84_Gravity_Implementation/2(lat_rad)  "lat"
  WGS84_2_ECEF/1(pE) -> WGS84_Gravity_Implementation/1(pE)  "pE"
  Compare To Constant/1 -> Assertion/1
  Interval Test/1 -> Assertion1/1
  Interval Test1/1 -> Assertion2/1

== system GRM_Airframe/GRM_Airframe/environment/atmosphere_static_ISO_2533 ==
  hBE : Inport
  env_glbl : Inport  Port=2
  Bus Creator1 : BusCreator  Inputs=6
  Bus Selector1 : BusSelector  OutputSignals=e_Tmp,e_pa
  Saturation : Saturate  UpperLimit=c_h_geope  LowerLimit=c_h_geop0
      settings: AttributesFormatString=|
      | %<UpperLimit>
      | %<LowerLimit>
  density : Subsystem
  geopot_height : Subsystem  mask{mean_earth_radius=c_r0}
      mask prompts: mean_earth_radius "Mean Earth Radius WGS 84 [m]"
      mask TypeOptions mean_earth_radius: mean_earth_radius/Value
  speed_of_sound : Subsystem
  tmp_and_pressure_ISO_2533 : Subsystem
  atm_stat : Outport
  wires:
  Saturation/1 -> tmp_and_pressure_ISO_2533/1(h_geop), Bus Creator1/2  "h_geop"
  hBE/1 -> geopot_height/1(hBE), Bus Creator1/1
  density/1(rho) -> Bus Creator1/5
  tmp_and_pressure_ISO_2533/2(pa) -> density/2(pa), Bus Creator1/6
  tmp_and_pressure_ISO_2533/1(Tmp) -> density/1(Tmp), Bus Creator1/4, speed_of_sound/1(Tmp)
  Bus Creator1/1 -> atm_stat/1  "atm_stat_bus"
  Bus Selector1/1 -> tmp_and_pressure_ISO_2533/2(e_Tmp)  "<e_Tmp>"
  geopot_height/1(h_geop) -> Saturation/1
  Bus Selector1/2 -> tmp_and_pressure_ISO_2533/3(e_pa)  "<e_pa>"
  env_glbl/1 -> Bus Selector1/1
  speed_of_sound/1(sos) -> Bus Creator1/3

== system GRM_Airframe/GRM_Airframe/environment/convert_to_local_frame ==
  gE : Inport
  Constant1 : Constant  Value=0
  Dot Product : DotProduct  InputSameDT=on  OutDataTypeStr=Inherit: Inherit via internal rule
  Sqrt : Sqrt  SaturateOnIntegerOverflow=on
  Vector Concatenate : Concatenate  NumInputs=3  Mode=Multidimensional array
  gBG : Outport
  wires:
  Dot Product/1 -> Sqrt/1
  Vector Concatenate/1 -> gBG/1  "gBG"
  Sqrt/1 -> Vector Concatenate/3
  Constant1/1 -> Vector Concatenate/1, Vector Concatenate/2
  gE/1 -> Dot Product/2, Dot Product/1

== system GRM_Airframe/GRM_Airframe/fin_actuators/Rudder ==
  siB_c : Inport
  tRRR : Inport  Port=2
  Add : Sum  Inputs=+-
  Add1 : Sum  Inputs=+-
  Add2 : Sum  Inputs=+++
  Constant : Constant  Value=unc_off
  Gain : Gain  Gain=omega^2
  Gain1 : Gain  Gain=unc_scale
  Gain2 : Gain  Gain=2*dmp*omega  Multiplication=Matrix(K*u)
  Gain3 : Gain  Gain=unc_bl
  Integrator : Integrator  ExternalReset=either  InitialCondition=d_siB_0
  Integrator1 : Integrator  InitialCondition=siB_0  LimitOutput=on  UpperSaturationLimit=siB_max  LowerSaturationLimit=siB_min  ShowSaturationPort=on
  Limiting_Acceleration : MATLAB Function  TreatAsAtomicUnit=on
  Limiting_Rate : MATLAB Function  TreatAsAtomicUnit=on
  Saturation : Saturate  UpperLimit=siB_max  LowerLimit=siB_min
  Saturation1 : Saturate  UpperLimit=siB_max  LowerLimit=siB_min
  Sign : Signum
  siB : Outport
  d_siB : Outport  Port=2
  dd_siB : Outport  Port=3
  wires:
  [siB] -> Limiting_Rate/1(siB)
  [siB] -> Limiting_Acceleration/1(siB)
  [d_siB] -> Limiting_Acceleration/2(d_siB)
  siB_c/1 -> Saturation/1  "siB_c"
  Constant/1 -> Add2/1
  Add2/1 -> Saturation1/1
  Saturation/1 -> Add/1
  Integrator/1 -> Gain2/1, Limiting_Rate/2(d_siB)  "d_siB"
  Limiting_Rate/1(d_siB_l) -> Integrator1/1, [d_siB], d_siB/1  "d_siB_l"
  Limiting_Acceleration/1(dd_siB_l) -> dd_siB/1, Integrator/1  "dd_siB_l"
  Add/1 -> Gain/1
  Gain/1 -> Add1/1
  Gain2/1 -> Add1/2
  Add1/1 -> Limiting_Acceleration/3(dd_siB)  "dd_siB"
  Integrator1/1 -> Add/2, Gain1/1  "siB"
  tRRR/1 -> Sign/1  "tRRR"
  Sign/1 -> Gain3/1
  Gain3/1 -> Add2/3
  Gain1/1 -> Add2/2
  Integrator1/2 -> Integrator/2  "sat"
  Saturation1/1 -> [siB], siB/1  "siB"

== system GRM_Airframe/GRM_Airframe/fin_actuators/Rudder1 ==
  siB_c : Inport
  tRRR : Inport  Port=2
  Add : Sum  Inputs=+-
  Add1 : Sum  Inputs=+-
  Add2 : Sum  Inputs=+++
  Constant : Constant  Value=unc_off
  Gain : Gain  Gain=omega^2
  Gain1 : Gain  Gain=unc_scale
  Gain2 : Gain  Gain=2*dmp*omega  Multiplication=Matrix(K*u)
  Gain3 : Gain  Gain=unc_bl
  Integrator : Integrator  ExternalReset=either  InitialCondition=d_siB_0
  Integrator1 : Integrator  InitialCondition=siB_0  LimitOutput=on  UpperSaturationLimit=siB_max  LowerSaturationLimit=siB_min  ShowSaturationPort=on
  Limiting_Acceleration : MATLAB Function  TreatAsAtomicUnit=on
  Limiting_Rate : MATLAB Function  TreatAsAtomicUnit=on
  Saturation : Saturate  UpperLimit=siB_max  LowerLimit=siB_min
  Saturation1 : Saturate  UpperLimit=siB_max  LowerLimit=siB_min
  Sign : Signum
  siB : Outport
  d_siB : Outport  Port=2
  dd_siB : Outport  Port=3
  wires:
  [siB] -> Limiting_Rate/1(siB)
  [siB] -> Limiting_Acceleration/1(siB)
  [d_siB] -> Limiting_Acceleration/2(d_siB)
  siB_c/1 -> Saturation/1  "siB_c"
  Constant/1 -> Add2/1
  Add2/1 -> Saturation1/1
  Saturation/1 -> Add/1
  Integrator/1 -> Gain2/1, Limiting_Rate/2(d_siB)  "d_siB"
  Limiting_Rate/1(d_siB_l) -> Integrator1/1, [d_siB], d_siB/1  "d_siB_l"
  Limiting_Acceleration/1(dd_siB_l) -> dd_siB/1, Integrator/1  "dd_siB_l"
  Add/1 -> Gain/1
  Gain/1 -> Add1/1
  Gain2/1 -> Add1/2
  Add1/1 -> Limiting_Acceleration/3(dd_siB)  "dd_siB"
  Integrator1/1 -> Add/2, Gain1/1  "siB"
  tRRR/1 -> Sign/1  "tRRR"
  Sign/1 -> Gain3/1
  Gain3/1 -> Add2/3
  Gain1/1 -> Add2/2
  Integrator1/2 -> Integrator/2  "sat"
  Saturation1/1 -> [siB], siB/1  "siB"

== system GRM_Airframe/GRM_Airframe/fin_actuators/Rudder2 ==
  siB_c : Inport
  tRRR : Inport  Port=2
  Add : Sum  Inputs=+-
  Add1 : Sum  Inputs=+-
  Add2 : Sum  Inputs=+++
  Constant : Constant  Value=unc_off
  Gain : Gain  Gain=omega^2
  Gain1 : Gain  Gain=unc_scale
  Gain2 : Gain  Gain=2*dmp*omega  Multiplication=Matrix(K*u)
  Gain3 : Gain  Gain=unc_bl
  Integrator : Integrator  ExternalReset=either  InitialCondition=d_siB_0
  Integrator1 : Integrator  InitialCondition=siB_0  LimitOutput=on  UpperSaturationLimit=siB_max  LowerSaturationLimit=siB_min  ShowSaturationPort=on
  Limiting_Acceleration : MATLAB Function  TreatAsAtomicUnit=on
  Limiting_Rate : MATLAB Function  TreatAsAtomicUnit=on
  Saturation : Saturate  UpperLimit=siB_max  LowerLimit=siB_min
  Saturation1 : Saturate  UpperLimit=siB_max  LowerLimit=siB_min
  Sign : Signum
  siB : Outport
  d_siB : Outport  Port=2
  dd_siB : Outport  Port=3
  wires:
  [siB] -> Limiting_Rate/1(siB)
  [siB] -> Limiting_Acceleration/1(siB)
  [d_siB] -> Limiting_Acceleration/2(d_siB)
  siB_c/1 -> Saturation/1  "siB_c"
  Constant/1 -> Add2/1
  Add2/1 -> Saturation1/1
  Saturation/1 -> Add/1
  Integrator/1 -> Gain2/1, Limiting_Rate/2(d_siB)  "d_siB"
  Limiting_Rate/1(d_siB_l) -> Integrator1/1, [d_siB], d_siB/1  "d_siB_l"
  Limiting_Acceleration/1(dd_siB_l) -> dd_siB/1, Integrator/1  "dd_siB_l"
  Add/1 -> Gain/1
  Gain/1 -> Add1/1
  Gain2/1 -> Add1/2
  Add1/1 -> Limiting_Acceleration/3(dd_siB)  "dd_siB"
  Integrator1/1 -> Add/2, Gain1/1  "siB"
  tRRR/1 -> Sign/1  "tRRR"
  Sign/1 -> Gain3/1
  Gain3/1 -> Add2/3
  Gain1/1 -> Add2/2
  Integrator1/2 -> Integrator/2  "sat"
  Saturation1/1 -> [siB], siB/1  "siB"

== system GRM_Airframe/GRM_Airframe/fin_actuators/Rudder3 ==
  siB_c : Inport
  tRRR : Inport  Port=2
  Add : Sum  Inputs=+-
  Add1 : Sum  Inputs=+-
  Add2 : Sum  Inputs=+++
  Constant : Constant  Value=unc_off
  Gain : Gain  Gain=omega^2
  Gain1 : Gain  Gain=unc_scale
  Gain2 : Gain  Gain=2*dmp*omega  Multiplication=Matrix(K*u)
  Gain3 : Gain  Gain=unc_bl
  Integrator : Integrator  ExternalReset=either  InitialCondition=d_siB_0
  Integrator1 : Integrator  InitialCondition=siB_0  LimitOutput=on  UpperSaturationLimit=siB_max  LowerSaturationLimit=siB_min  ShowSaturationPort=on
  Limiting_Acceleration : MATLAB Function  TreatAsAtomicUnit=on
  Limiting_Rate : MATLAB Function  TreatAsAtomicUnit=on
  Saturation : Saturate  UpperLimit=siB_max  LowerLimit=siB_min
  Saturation1 : Saturate  UpperLimit=siB_max  LowerLimit=siB_min
  Sign : Signum
  siB : Outport
  d_siB : Outport  Port=2
  dd_siB : Outport  Port=3
  wires:
  [siB] -> Limiting_Rate/1(siB)
  [siB] -> Limiting_Acceleration/1(siB)
  [d_siB] -> Limiting_Acceleration/2(d_siB)
  siB_c/1 -> Saturation/1  "siB_c"
  Constant/1 -> Add2/1
  Add2/1 -> Saturation1/1
  Saturation/1 -> Add/1
  Integrator/1 -> Gain2/1, Limiting_Rate/2(d_siB)  "d_siB"
  Limiting_Rate/1(d_siB_l) -> Integrator1/1, [d_siB], d_siB/1  "d_siB_l"
  Limiting_Acceleration/1(dd_siB_l) -> dd_siB/1, Integrator/1  "dd_siB_l"
  Add/1 -> Gain/1
  Gain/1 -> Add1/1
  Gain2/1 -> Add1/2
  Add1/1 -> Limiting_Acceleration/3(dd_siB)  "dd_siB"
  Integrator1/1 -> Add/2, Gain1/1  "siB"
  tRRR/1 -> Sign/1  "tRRR"
  Sign/1 -> Gain3/1
  Gain3/1 -> Add2/3
  Gain1/1 -> Add2/2
  Integrator1/2 -> Integrator/2  "sat"
  Saturation1/1 -> [siB], siB/1  "siB"

== system GRM_Airframe/GRM_Airframe/fin_actuators/control_allocation ==
  siB : Inport
  d_siB : Inport  Port=2
  dd_siB : Inport  Port=3
  Constant8 : Constant  Value=Tr3r4
  Product : Product  Multiplication=Matrix(*)
  Product1 : Product  Multiplication=Matrix(*)
  Product2 : Product  Multiplication=Matrix(*)
  Tr3r4 : Outport
  finB : Outport  Port=2
  d_finB : Outport  Port=3
  dd_finB : Outport  Port=4
  wires:
  Product2/1 -> dd_finB/1  "dd_afinB"
  dd_siB/1 -> Product2/2
  Product1/1 -> d_finB/1  "d_afinB"
  d_siB/1 -> Product1/2
  siB/1 -> Product/2
  Constant8/1 -> Product/1, Product1/1, Product2/1, Tr3r4/1  "Tr3r4"
  Product/1 -> finB/1  "afinB"

== system GRM_Airframe/GRM_Airframe/gravity/launch_rail ==
  gBG_c : Inport
  hBE : Inport  Port=2
  Constant1 : Constant  Value=flag_I_gravity_switch
  Constant3 : Constant  Value=0
  Subtract : Sum  Inputs=++-
  Switch : Switch  Criteria=u2 > Threshold  Threshold=0.05
  Vector Concatenate : Concatenate  NumInputs=3
  initial_altitude : Subsystem
  gBG : Outport
  wires:
  initial_altitude/1(hBE_0) -> Subtract/3
  gBG_c/1 -> Switch/1
  Vector Concatenate/1 -> Switch/3
  Switch/1 -> gBG/1  "gBG"
  Constant3/1 -> Vector Concatenate/3, Vector Concatenate/2, Vector Concatenate/1
  Subtract/1 -> Switch/2
  hBE/1 -> Subtract/1
  Constant1/1 -> Subtract/2

== system GRM_Airframe/GRM_Airframe/motion_kinematics/calc_motion_kinematics ==
  lat : Inport
  lon : Inport  Port=2
  qIB : Inport  Port=3
  calc_transformation_matrix : Subsystem
  earth_rotation : Subsystem
  wIEE : Outport
  TIE : Outport  Port=2
  TEB : Outport  Port=3
  TGB : Outport  Port=4
  TEG : Outport  Port=5
  wEGG : Outport  Port=6
  TIB : Outport  Port=7
  wires:
  calc_transformation_matrix/3(TIB) -> TIB/1
  calc_transformation_matrix/2(TGB) -> TGB/1
  calc_transformation_matrix/1(TEB) -> TEB/1
  qIB/1 -> calc_transformation_matrix/3(qIB)
  earth_rotation/4(qEG) -> calc_transformation_matrix/2(qEG)
  earth_rotation/3(qIE) -> calc_transformation_matrix/1(qIE)
  lat/1 -> earth_rotation/1(lat)
  lon/1 -> earth_rotation/2(lon)
  earth_rotation/6(wEGG) -> wEGG/1
  earth_rotation/5(TEG) -> TEG/1
  earth_rotation/2(TIE) -> TIE/1
  earth_rotation/1(wIEE) -> wIEE/1

== system GRM_Airframe/GRM_Airframe/propulsion/prp_look_up ==
  env_glbl_bus : Inport
  Bus Selector1 : BusSelector  OutputSignals=T_sim_glbl,T_sim_lnch
  Constant : Constant  Value=0
  Constant1 : Constant  Value=0
  Saturation : Saturate  UpperLimit=t_prp1(end)  LowerLimit=0
      settings: AttributesFormatString=|
      | %<UpperLimit>
      | %<LowerLimit>
  Subtract : Sum  Inputs=+-
  Switch : Switch  Criteria=u2 > Threshold
  Switch1 : Switch  Criteria=u2 > Threshold
  Switch2 : Switch  Criteria=u2 > Threshold
  Vector Concatenate : Concatenate  NumInputs=3
  mass_flow_lookup : Lookup_n-D  NumberOfTableDimensions=1  BreakpointsForDimension1=t_dmB  Table=d_mB_lookup  ExtrapMethod=Clip  UseLastTableValue=on  InternalRulePriority=Speed  RndMeth=Simplest  InputSameDT=on
  thrust_lookup : Lookup_n-D  NumberOfTableDimensions=1  BreakpointsForDimension1=t_prp1  Table=F_prp  ExtrapMethod=Clip  UseLastTableValue=on  InternalRulePriority=Speed  RndMeth=Simplest  InputSameDT=on
  dmB : Outport
  FBPM : Outport  Port=2
  wires:
  Switch2/1 -> dmB/1  "dmB"
  mass_flow_lookup/1 -> Switch2/1
  Switch1/1 -> Vector Concatenate/1  "a_FBPM"
  Constant1/1 -> Vector Concatenate/2, Vector Concatenate/3
  Vector Concatenate/1 -> FBPM/1  "FBPM"
  Saturation/1 -> thrust_lookup/1, Switch2/3, Switch2/2, mass_flow_lookup/1
  Subtract/1 -> Switch/2, Switch/1
  Constant/1 -> Switch/3
  env_glbl_bus/1 -> Bus Selector1/1
  Bus Selector1/1 -> Subtract/1  "<T_sim_glbl>"
  thrust_lookup/1 -> Switch1/1
  Switch/1 -> Switch1/3, Switch1/2, Saturation/1
  Bus Selector1/2 -> Subtract/2  "<T_sim_lnch>"

== system GRM_Airframe/GRM_Airframe/propulsion/prp_uncertainty ==
  FBPM : Inport
  wab : Inport  Port=2
  3_rot_mat : Subsystem  mask(Rotation um 1, 2 oder 3 Achsen){rot_1=Rotation um z-Achse, rot_2=Rotation um y-Achse, rot_3=Rotation um x-Achse}
      mask prompts: rot_1 "1. Rotation"; rot_2 "2. Rotation"; rot_3 "3. Rotation"
      mask help:
      | Dieser Block liefert die Rotationsmatrix T12 für den Fall zurück, dass sich das Ziel-Koordinatensystem (1) durch Drehungen um 1, 2 oder 3 Achsen gegenüber dem Ausgangskoordinatensystem (2) beschreiben lässt (passive Drehung).
      |
      | Die Anzahl der Rotation sowie die Reihenfolge ist frei einstellbar.
      |
      | Die Rotationswinkel haben die Einheit [rad].
      mask TypeOptions rot_1: Rotation um x-Achse | Rotation um y-Achse | Rotation um z-Achse
      mask TypeOptions rot_2: Rotation um x-Achse | Rotation um y-Achse | Rotation um z-Achse
      mask TypeOptions rot_3: Rotation um x-Achse | Rotation um y-Achse | Rotation um z-Achse
  Bus Selector : BusSelector  OutputSignals=pBSB
  Product : Product  Multiplication=Matrix(*)
  Product1 : Product
  Subtract : Sum  Inputs=+-
  Thrust_rot_z : Constant  Value=unc_prp_z
  cross_product : Subsystem
      mask help: cross product r3 = r1 x r2
      mask Help:
      | Name:
      | 
      |     cross_product
      | 
      | Description:
      | 
      |     This block implements the cross product r3 = r1 x r2.
      | 
      | Inputs  [size] [data type] [unit]:
      | 
      |     vector 1  [3] [double] [-]
      |     vector 2  [3] [double] [-]
      | 
      | Outputs  [size] [data type] [unit]:
      | 
      |     resulting vector  [3] [double] [-]
      mask Display: disp(' r3 = r1 x r2')
  pNPB : Constant  Value=pNPB
  thrust_rot_x : Constant  Value=unc_prp_x
  thrust_rot_y : Constant  Value=unc_prp_y
  uncert_thrust : Constant  Value=unc_prp_scale
  FBPB : Outport
  MBPB : Outport  Port=2
  wires:
  Subtract/1 -> cross_product/1(r1)
  pNPB/1 -> Subtract/2
  Product1/1 -> Product/2
  uncert_thrust/1 -> Product1/2
  Bus Selector/1 -> Subtract/1  "<pBSB>"
  wab/1 -> Bus Selector/1
  cross_product/1(r1_x_r2) -> MBPB/1  "MBPB"
  thrust_rot_y/1 -> 3_rot_mat/2(wi2)
  3_rot_mat/1(T12) -> Product/1
  FBPM/1 -> Product1/1
  Product/1 -> FBPB/1, cross_product/2(r2)  "FBPB"
  thrust_rot_x/1 -> 3_rot_mat/3(wi3)
  Thrust_rot_z/1 -> 3_rot_mat/1(wi1)

== system GRM_Airframe/GRM_Airframe/rb_eom/calc_bus_flight_dyn_bus_entries ==
  mot_kin : Inport
  eom : Inport  Port=2
  Bus Selector : BusSelector  OutputSignals=pBII,vBII,qIB,wBIB,d_wBIB,d_vBII
  Bus Selector3 : BusSelector  OutputSignals=TIB,TIE
  Math Function : Math  Operator=transpose  SaturateOnIntegerOverflow=on
  Product : Product  Multiplication=Matrix(*)
  Product1 : Product  Multiplication=Matrix(*)
  Subsystem2 : Subsystem
  quaternion_to_euler_angles : Subsystem
      mask help: transforms quaternions to Euler angles (roll, pitch, yaw)
      mask Help:
      | Name:
      | 
      |     quaternion_to_euler_angles
      | 
      | Description:
      | 
      |     This block implements the transformation of a quaternion into the
      |     corresponding Euler angles (zyx-sequence, roll, pitch, yaw).
      | 
      | Inputs  [size] [data type] [unit]:
      | 
      |     quaternion  [4] [double] [-]
      | 
      | Outputs  [size] [data type] [unit]:
      | 
      |     roll angle phi  [1] [double] [rad]
      |     pitch angle theta  [1] [double] [rad]
      |     yaw angle psi  [1] [double] [rad]
      mask Display:
      | %disp (' q --> (Phi,Theta,Psi) [rad]')
      | disp('q \rightarrow eu(\Phi;\Theta;\Psi)','texmode','on')
  aBIB : Outport
  lon : Outport  Port=2
  lat : Outport  Port=3
  hBE : Outport  Port=4
  vBII : Outport  Port=5
  qIB : Outport  Port=6
  wBIB : Outport  Port=7
  d_wBIB : Outport  Port=8
  d_vBII : Outport  Port=9
  pBII : Outport  Port=10
  euIB : Outport  Port=11
  vBIB : Outport  Port=12
  wires:
  Product1/1 -> vBIB/1  "vBIB"
  quaternion_to_euler_angles/1(eulx) -> euIB/1  "euIB"
  Bus Selector/5 -> d_wBIB/1  "<d_wBIB>"
  Bus Selector/4 -> wBIB/1  "<wBIB>"
  Bus Selector/3 -> qIB/1, quaternion_to_euler_angles/1(q)  "<qIB>"
  Bus Selector/2 -> vBII/1, Product1/2  "<vBII>"
  Subsystem2/3(hBE) -> hBE/1  "hBE"
  Subsystem2/2(lat) -> lat/1
  Subsystem2/1(lon) -> lon/1
  Product/1 -> aBIB/1  "aBIB"
  Bus Selector/6 -> d_vBII/1, Product/2  "<d_vBII>"
  Bus Selector3/1 -> Math Function/1  "<TIB>"
  Math Function/1 -> Product/1, Product1/1  "TBI"
  eom/1 -> Bus Selector/1
  Bus Selector3/2 -> Subsystem2/1(TIE)  "<TIE>"
  mot_kin/1 -> Bus Selector3/1
  Bus Selector/1 -> Subsystem2/2(pBII), pBII/1  "<pBII>"

== system GRM_Airframe/GRM_Airframe/rb_eom/eom_6dof ==
  for_mom : Inport
  wab : Inport  Port=2
  Bus Selector1 : BusSelector  OutputSignals=mB,JBBB
  Bus Selector2 : BusSelector  OutputSignals=FBTB,MBTB
  Constant : Constant  Value=[pBII_0; vBII_0; qIB_0; wBIB_0]
  Constant9 : Constant  Value=[0 0 0; 0 0 0; 0 0 0]
  Rigid_Body_EOM_6_DOF : Subsystem  mask{flag_Kraft=FBTB}
      mask prompts: flag_Kraft "Input Kraftvektor"
      mask help:
      | 6DOF-Bewegungsgleichungen im ECI-System mit
      | zeitvariantem Massenträgheitsmoment.
      |
      | Modell Varianten:
      | - Koordinatensystem des Kraftvektor:
      |      FBTI : Inertial System I
      |      FBTB : Körperfestes System B
      mask init:
      | switch flag_Kraft
      |     case 1
      |         port_label_kraft = 'FBTI';
      |     case 2
      |         port_label_kraft = 'FBTB';
      | end
      mask TypeOptions flag_Kraft: FBTI | FBTB
      mask DialogControl Container4 Prompt: Modell Einstellungen
      mask Display:
      | port_label ('input',1,port_label_kraft )
      | port_label ('input',2,'MBTB' )
      | port_label ('input',3,'mB' )
      | port_label ('input',4,'x0' )
      | port_label ('input',5,'JBB' )
      | port_label ('input',6,'d_JBB' )
      | port_label ('output',1,'rb_eom' )
  eom : Outport
  wires:
  wab/1 -> Bus Selector1/1
  Bus Selector1/1 -> Rigid_Body_EOM_6_DOF/3(mB)  "<mB>"
  Constant/1 -> Rigid_Body_EOM_6_DOF/4(x0)
  for_mom/1 -> Bus Selector2/1
  Bus Selector1/2 -> Rigid_Body_EOM_6_DOF/5(JBB)  "<JBBB>"
  Constant9/1 -> Rigid_Body_EOM_6_DOF/6(d_JBB)
  Rigid_Body_EOM_6_DOF/1(rb_eom) -> eom/1
  Bus Selector2/1 -> Rigid_Body_EOM_6_DOF/1(FBTX)  "<FBTB>"
  Bus Selector2/2 -> Rigid_Body_EOM_6_DOF/2(MBTB)  "<MBTB>"

== system GRM_Airframe/GRM_Airframe/stream_flow/calc_stream_flow ==
  TIB : Inport
  wIEE : Inport  Port=2
  TIE : Inport  Port=3
  TGB : Inport  Port=4
  vBII : Inport  Port=5
  pBII : Inport  Port=6
  wBIB : Inport  Port=7
  rho : Inport  Port=8
  sos : Inport  Port=9
  hBE : Inport  Port=10
  vWEG : Inport  Port=11
  Bus Creator : BusCreator  Inputs=9
  Math Function : Math  Operator=transpose  SaturateOnIntegerOverflow=on
  Math Function1 : Math  Operator=transpose  SaturateOnIntegerOverflow=on
  Product : Product  Multiplication=Matrix(*)
  Product1 : Product  Multiplication=Matrix(*)
  Subsystem1 : Subsystem
  velocity_vector_transformation : Subsystem
  str_flow : Outport
  wires:
  Product1/1 -> Subsystem1/1(vWEB)  "vBEB_w"
  Math Function1/1 -> Product1/1  "TBG"
  vWEG/1 -> Product1/2
  TGB/1 -> Math Function1/1
  pBII/1 -> velocity_vector_transformation/4(pBII)
  TIB/1 -> Math Function/1
  rho/1 -> Subsystem1/4(rho)
  sos/1 -> Subsystem1/5(sos)
  hBE/1 -> Bus Creator/9
  wBIB/1 -> Subsystem1/3(wBIB)
  Bus Creator/1 -> str_flow/1  "str_flow_bus"
  wIEE/1 -> velocity_vector_transformation/1(wIEE)
  Subsystem1/1(al) -> Bus Creator/1  "alB"
  Subsystem1/7(th) -> Bus Creator/7  "inB"
  velocity_vector_transformation/1(vBEI) -> Product/2
  Subsystem1/3(qdynB) -> Bus Creator/3
  TIE/1 -> velocity_vector_transformation/2(TIE)
  Subsystem1/6(wBIB_star) -> Bus Creator/6
  Product/1 -> Subsystem1/2(vBEB)  "vBEB_k"
  Subsystem1/5(a_vB) -> Bus Creator/5
  vBII/1 -> velocity_vector_transformation/3(vBII)
  Subsystem1/8(fi) -> Bus Creator/8  "fiB"
  Subsystem1/2(be) -> Bus Creator/2  "beB"
  Math Function/1 -> Product/1  "TBI"
  Subsystem1/4(MaB) -> Bus Creator/4

== system GRM_Airframe/GRM_Airframe/weight_and_balance/center_of_gravity ==
  mB : Inport
  mM : Inport  Port=2
  Add{,1..5} (6 alike) : Sum
  Constant : Constant  Value=m0
  Constant1 : Constant  Value=unc_cg_y
  Constant2 : Constant  Value=unc_cg_z
  Constant3 : Constant  Value=unc_cg_x
  Constant4 : Constant  Value=xMPB
  Constant5 : Constant  Value=y0PB
  Constant6 : Constant  Value=x0PB
  Constant7 : Constant  Value=yMPB
  Constant8 : Constant  Value=z0PB
  Constant9 : Constant  Value=zMPB
  Divide : Product  Inputs=/*
  Divide1 : Product  Inputs=/*
  Divide2 : Product  Inputs=/*
  Product{,1..5} (6 alike) : Product
  Vector Concatenate : Concatenate  NumInputs=3
  pBSB : Outport
  wires:
  Constant4/1 -> Product1/2  "xMPB"
  Constant5/1 -> Product2/2  "y0PB"
  Constant6/1 -> Product/2  "x0PB"
  Constant7/1 -> Product3/2  "yMPB"
  Constant8/1 -> Product4/2  "z0PB"
  Constant9/1 -> Product5/2  "zMPB"
  Add4/1 -> Vector Concatenate/1
  Add3/1 -> Vector Concatenate/2
  Add5/1 -> Vector Concatenate/3
  Divide1/1 -> Add3/1
  Divide/1 -> Add4/1
  Constant3/1 -> Add4/2
  Constant1/1 -> Add3/2
  Constant2/1 -> Add5/2
  Divide2/1 -> Add5/1
  Vector Concatenate/1 -> pBSB/1  "pBSB"
  Add2/1 -> Divide2/2
  Product4/1 -> Add2/2
  Product5/1 -> Add2/1
  Add1/1 -> Divide1/2
  Product2/1 -> Add1/2
  Product3/1 -> Add1/1
  mB/1 -> Divide/1, Divide1/1, Divide2/1
  Add/1 -> Divide/2
  mM/1 -> Product1/1, Product3/1, Product5/1
  Product/1 -> Add/2
  Product1/1 -> Add/1
  Constant/1 -> Product/1, Product2/1, Product4/1
